simulink model "hmag_ctrl_with_hcomp_2021_09_27"  (R2020a)
settings: Solver=ode23tb  StartTime=0.0  StopTime=simlength  MaxStep=Ts
values from neighbouring files (symbols this model uses):
  Afd = [exp(-Ts*w)*(1+Ts*w) exp(-Ts*w)*Ts; -exp(-Ts*w)*Ts*w^2 exp(-Ts*w)*(1-Ts*w)]    [init_2021_09_27.m]
  Afd_res = [exp(-Ts*wres)*(1+Ts*wres) exp(-Ts*wres)*Ts; -exp(-Ts*wres)*Ts*wres^2 exp(-Ts*wres)*(1-Ts*wres)]    [init_2021_09_27.m]
  Ares = 1    [init_2021_09_27.m]
  Bfd = [(1-exp(-Ts*w)*(1+Ts*w))/w^2 exp(-Ts*w)*Ts]'    [init_2021_09_27.m]
  Bfd_res = [(1-exp(-Ts*wres)*(1+Ts*wres))/wres^2 exp(-Ts*wres)*Ts]'    [init_2021_09_27.m]
  Cf = [2*w^2 0]    [init_2021_09_27.m]
  Cf_res = [2*wres^2 0]    [init_2021_09_27.m]
  ki = 2    [init_2021_09_27.m]
  ki_comp = 2e-1    (= 0.2)    [init_2021_09_27.m]
  kp = 1    [init_2021_09_27.m]
  kp_comp = 1e-1    (= 0.1)    [init_2021_09_27.m]
  pll_i1 = 2*pi/wres    (= 0.00507614213198)    [init_2021_09_27.m]
  pll_p = 2*pi/wres    (= 0.00507614213198)    [init_2021_09_27.m]
  q1kalman = Ts*10    (= 0.0005)    [init_2021_09_27.m]
  q1kalman_res = Ts    (= 5e-05)    [init_2021_09_27.m]
  q2kalman = Ts*10    (= 0.0005)    [init_2021_09_27.m]
  q2kalman_res = Ts    (= 5e-05)    [init_2021_09_27.m]
  Rkalman = 1e-2/q1kalman    (= 20)    [init_2021_09_27.m]
  Rkalman_res = 1/Ts    (= 20000)    [init_2021_09_27.m]
  simlength = 50    [init_2021_09_27.m]
  Tc = 1e-5    (= 1e-05)    [init_2021_09_27.m]
  Ts = 1/20e3    (= 5e-05)    [init_2021_09_27.m]
  w = 2*pi*f    (= 314.159265359)    [init_2021_09_27.m]
  wres = 197*2*pi    (= 1237.78750551)    [init_2021_09_27.m]
undefined symbols (not defined in the file or in its folder): magnitude
libraries: simulink x1, cstblocks x1
settings Model: SimulationMode=accelerator  Creator=dbagn  LastModifiedBy=dabagnara
settings SolverCC: SolverResetMethod=Robust
settings DataIOCC: ReturnWorkspaceOutputs=off

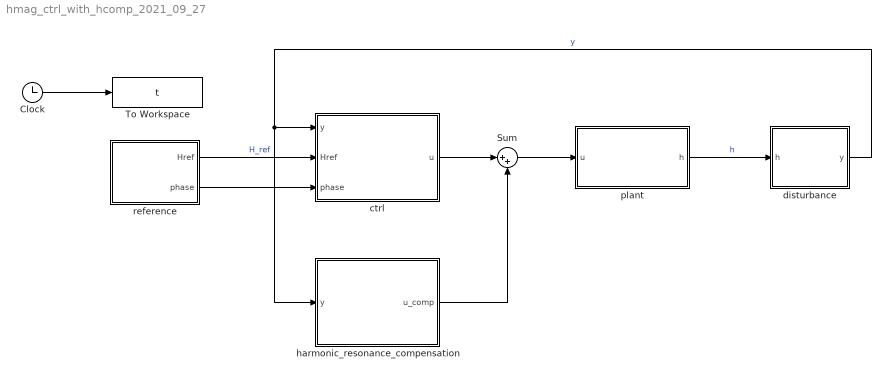
== system hmag_ctrl_with_hcomp_2021_09_27 ==
  Clock : Clock
  Sum : Sum  Inputs=|++
  To Workspace : ToWorkspace  VariableName=t  SampleTime=Tc
      settings: MaxDataPoints=Nc
  ctrl : Subsystem
  disturbance : Subsystem
  harmonic_resonance_compensation : Subsystem
  plant : Subsystem
  reference : Subsystem
  wires:
  reference/1(Href) -> ctrl/2(Href)  "H_ref"
  plant/1(h) -> disturbance/1(h)  "h"
  disturbance/1(y) -> harmonic_resonance_compensation/1(y), ctrl/1(y)  "y"
  reference/2(phase) -> ctrl/3(phase)
  Clock/1 -> To Workspace/1
  ctrl/1(u) -> Sum/1
  Sum/1 -> plant/1(u)
  harmonic_resonance_compensation/1(u_comp) -> Sum/2

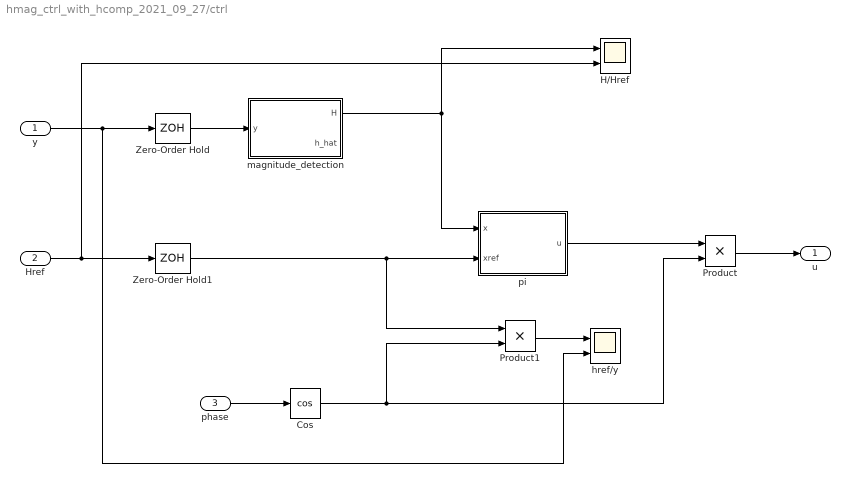
== system hmag_ctrl_with_hcomp_2021_09_27/ctrl ==
  y : Inport
  Href : Inport  Port=2
  phase : Inport  Port=3
  Cos : Trigonometry  Operator=cos
  H/Href : Scope  NumInputPorts=2
  Product : Product
  Product1 : Product
  Zero-Order Hold : ZeroOrderHold  SampleTime=Ts
  Zero-Order Hold1 : ZeroOrderHold  SampleTime=Ts
  href/y : Scope  NumInputPorts=2
  magnitude_detection : Subsystem
  pi : Subsystem  mask{kp=kp, ki=ki, ts=Ts, sat_pos=inf, sat_neg=-inf}
  u : Outport  VectorParamsAs1DForOutWhenUnconnected=off
  wires:
  Href/1 -> H/Href/2, Zero-Order Hold1/1
  y/1 -> href/y/2, Zero-Order Hold/1
  magnitude_detection/1(H) -> H/Href/1, pi/1(x)
  Zero-Order Hold/1 -> magnitude_detection/1(y)
  Zero-Order Hold1/1 -> pi/2(xref), Product1/1
  phase/1 -> Cos/1
  Cos/1 -> Product/2, Product1/2
  Product/1 -> u/1
  Product1/1 -> href/y/1
  pi/1(u) -> Product/1

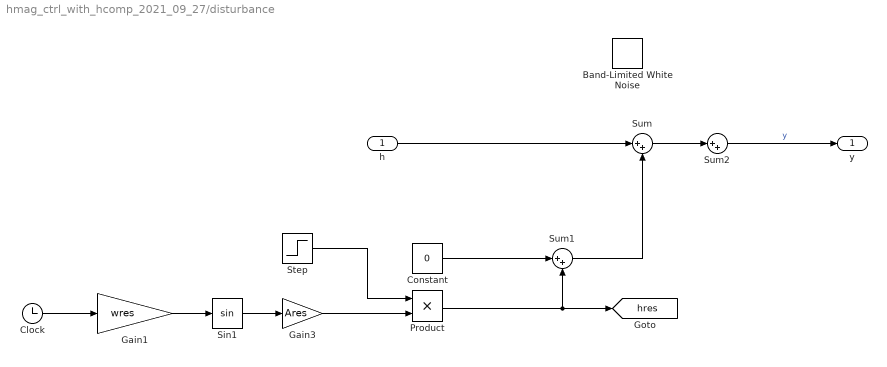
== system hmag_ctrl_with_hcomp_2021_09_27/disturbance ==
  h : Inport
  Band-Limited White Noise : simulink/Sources/Band-Limited White Noise  Cov=Tc  Ts=Tc  seed=[23341]
  Clock : Clock
  Constant : Constant  Value=0
  Gain1 : Gain  Gain=wres
  Gain3 : Gain  Gain=Ares
  Product : Product
  Sin1 : Trigonometry
  Step : Step  Time=simlength/2  Before=1  SampleTime=0
  Sum : Sum  Inputs=|++
  Sum1 : Sum  Inputs=|++
  Sum2 : Sum  Inputs=|++
  y : Outport
  tag scope: hres=global
  wires:
  Sin1/1 -> Gain3/1
  Clock/1 -> Gain1/1
  Sum/1 -> Sum2/1
  Constant/1 -> Sum1/1
  Sum2/1 -> y/1  "y"
  Sum1/1 -> Sum/2
  Gain1/1 -> Sin1/1
  h/1 -> Sum/1
  Gain3/1 -> Product/2
  Step/1 -> Product/1
  Product/1 -> Sum1/2, [hres]

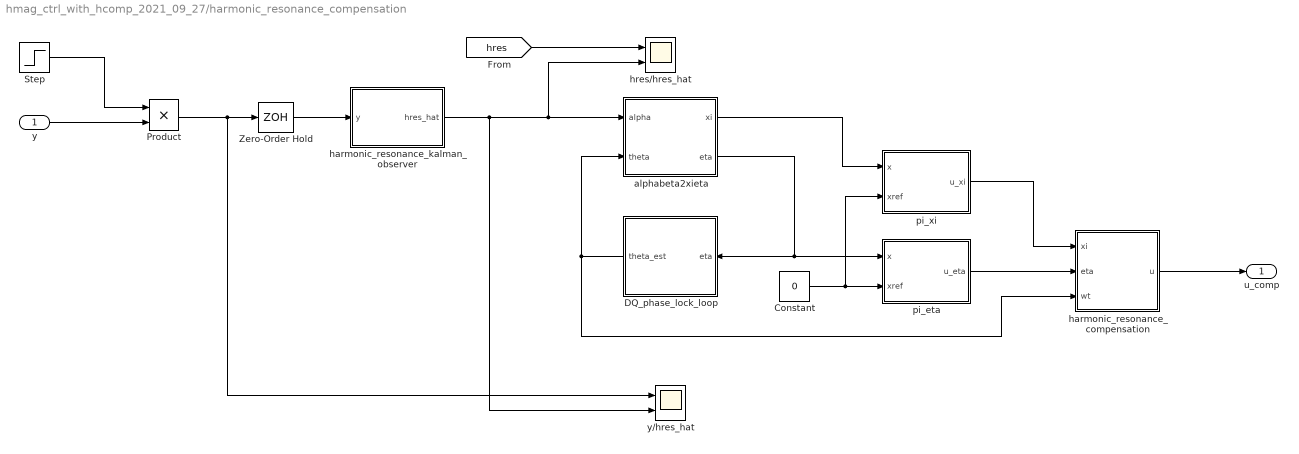
== system hmag_ctrl_with_hcomp_2021_09_27/harmonic_resonance_compensation ==
  y : Inport
  Constant : Constant  Value=0
  DQ_phase_lock_loop : Subsystem
  Product : Product
  Step : Step  Time=simlength/2  SampleTime=0
  Zero-Order Hold : ZeroOrderHold  SampleTime=Ts
  alphabeta2xieta : Subsystem
  harmonic_resonance_compensation : Subsystem
  harmonic_resonance_kalman_observer : Subsystem
  hres/hres_hat : Scope  NumInputPorts=2
  "pi_eta " : Subsystem  mask{kp=kp_comp, ki=ki_comp, ts=Ts, sat_pos=inf, sat_neg=-inf}
  pi_xi : Subsystem  mask{kp=kp_comp, ki=ki_comp, ts=Ts, sat_pos=inf, sat_neg=-inf}
  y/hres_hat : Scope  NumInputPorts=2
  u_comp : Outport  VectorParamsAs1DForOutWhenUnconnected=off
  wires:
  Zero-Order Hold/1 -> harmonic_resonance_kalman_observer/1(y)
  Constant/1 -> pi_xi/2(xref), "pi_eta "/2(xref)
  harmonic_resonance_kalman_observer/1(hres_hat) -> y/hres_hat/2, hres/hres_hat/2, alphabeta2xieta/1(alpha)
  pi_xi/1(u_xi) -> harmonic_resonance_compensation/1(xi)
  "pi_eta "/1(u_eta) -> harmonic_resonance_compensation/2(eta)
  alphabeta2xieta/2(eta) -> "pi_eta "/1(x), DQ_phase_lock_loop/1(eta)
  DQ_phase_lock_loop/1(theta_est) -> harmonic_resonance_compensation/3(wt), alphabeta2xieta/2(theta)
  alphabeta2xieta/1(xi) -> pi_xi/1(x)
  [hres] -> hres/hres_hat/1
  harmonic_resonance_compensation/1(u) -> u_comp/1
  Step/1 -> Product/1
  y/1 -> Product/2
  Product/1 -> y/hres_hat/1, Zero-Order Hold/1

== system hmag_ctrl_with_hcomp_2021_09_27/plant ==
  u : Inport
  LTI System : cstblocks/LTI System  sys=plant  IC=[]
  h : Outport  VectorParamsAs1DForOutWhenUnconnected=off
  wires:
  LTI System/1 -> h/1
  u/1 -> LTI System/1

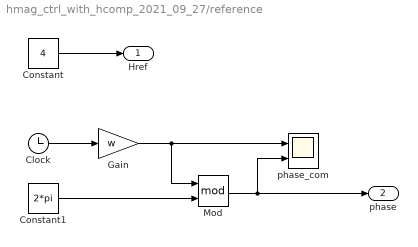
== system hmag_ctrl_with_hcomp_2021_09_27/reference ==
  Clock : Clock
  Constant : Constant  Value=4
  Constant1 : Constant  Value=2*pi
  Gain : Gain  Gain=w
  Mod : Math  Operator=mod  SaturateOnIntegerOverflow=on
  phase_com : Scope  NumInputPorts=2
  Href : Outport
  phase : Outport  Port=2
  wires:
  Clock/1 -> Gain/1
  Constant/1 -> Href/1
  Constant1/1 -> Mod/2
  Gain/1 -> phase_com/1, Mod/1
  Mod/1 -> phase_com/2, phase/1

== system hmag_ctrl_with_hcomp_2021_09_27/ctrl/magnitude_detection ==
  y : Inport
  Manual Switch : ManualSwitch
  kalman observer : Subsystem  Commented=on
  magnitude_calc : Subsystem
  H : Outport
  h_hat : Outport  Port=2
  wires:
  magnitude_calc/1(a) -> H/1
  y/1 -> Manual Switch/1, kalman observer/1(y)
  Manual Switch/1 -> h_hat/1, magnitude_calc/1(alpha)
  kalman observer/1(h_hat) -> Manual Switch/2

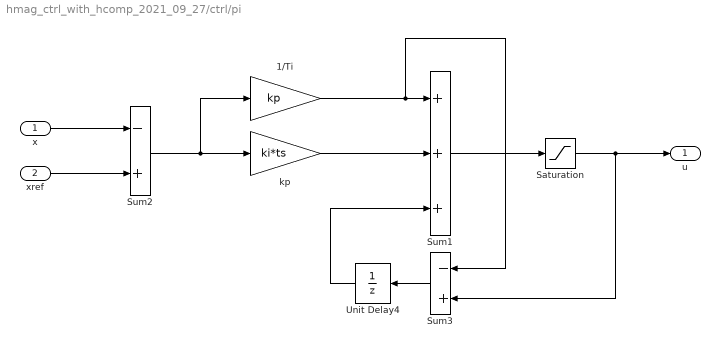
== system hmag_ctrl_with_hcomp_2021_09_27/ctrl/pi ==
  x : Inport
  xref : Inport  Port=2
  1/Ti : Gain  Gain=kp  SaturateOnIntegerOverflow=on  OutDataTypeStr=Inherit: Same as input  ParamDataTypeStr=Inherit: Same as input
  Saturation : Saturate  UpperLimit=sat_pos  LowerLimit=sat_neg
  Sum1 : Sum  Inputs=+++  SaturateOnIntegerOverflow=on
  Sum2 : Sum  Inputs=-+  SaturateOnIntegerOverflow=on
  Sum3 : Sum  Inputs=-+  SaturateOnIntegerOverflow=on
  Unit Delay4 : UnitDelay  SampleTime=ts  HasFrameUpgradeWarning=on
  kp : Gain  Gain=ki*ts  SaturateOnIntegerOverflow=on  OutDataTypeStr=Inherit: Same as input  ParamDataTypeStr=Inherit: Same as input
  u : Outport
  wires:
  xref/1 -> Sum2/2
  kp/1 -> Sum1/2
  Sum2/1 -> kp/1, 1/Ti/1
  1/Ti/1 -> Sum1/1, Sum3/1
  Sum3/1 -> Unit Delay4/1
  x/1 -> Sum2/1
  Sum1/1 -> Saturation/1
  Unit Delay4/1 -> Sum1/3
  Saturation/1 -> u/1, Sum3/2

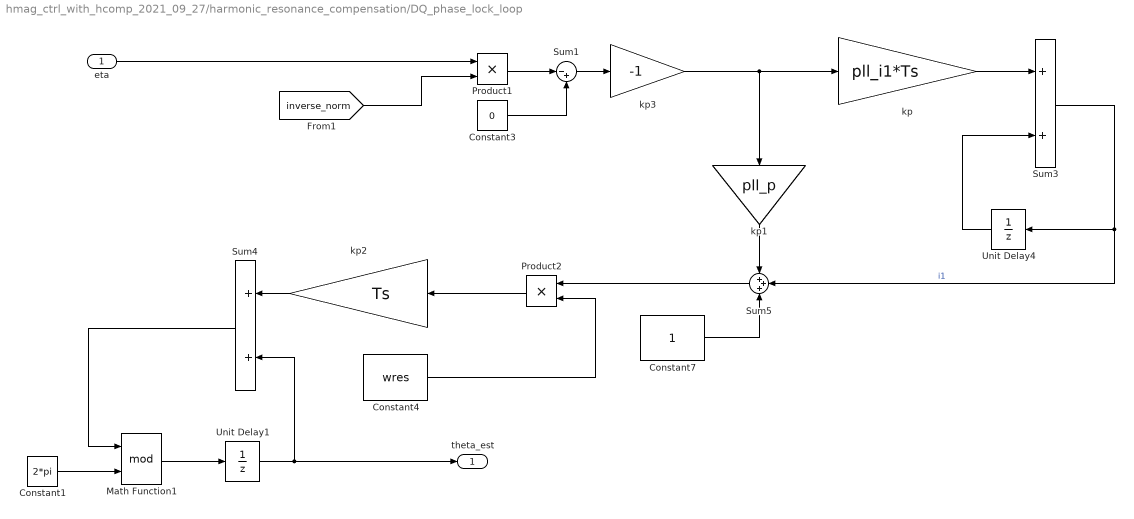
== system hmag_ctrl_with_hcomp_2021_09_27/harmonic_resonance_compensation/DQ_phase_lock_loop ==
  eta : Inport
  Constant1 : Constant  Value=2*pi
  Constant3 : Constant  Value=0
  Constant4 : Constant  Value=wres
  Constant7 : Constant
  Math Function1 : Math  Operator=mod  SignedPower=on  SaturateOnIntegerOverflow=on
  Product1 : Product  RndMeth=Zero
  Product2 : Product  RndMeth=Zero
  Sum1 : Sum  Inputs=|-+
  Sum3 : Sum  SaturateOnIntegerOverflow=on
  Sum4 : Sum  SaturateOnIntegerOverflow=on
  Sum5 : Sum  Inputs=+++
  Unit Delay1 : UnitDelay  SampleTime=Ts  HasFrameUpgradeWarning=on
  Unit Delay4 : UnitDelay  SampleTime=Ts  HasFrameUpgradeWarning=on
  kp : Gain  Gain=pll_i1*Ts  SaturateOnIntegerOverflow=on  OutDataTypeStr=Inherit: Same as input  ParamDataTypeStr=Inherit: Same as input
  kp1 : Gain  Gain=pll_p  SaturateOnIntegerOverflow=on  OutDataTypeStr=Inherit: Same as input  ParamDataTypeStr=Inherit: Same as input
  kp2 : Gain  Gain=Ts  SaturateOnIntegerOverflow=on  OutDataTypeStr=Inherit: Same as input  ParamDataTypeStr=Inherit: Same as input
  kp3 : Gain  Gain=-1  SaturateOnIntegerOverflow=on  OutDataTypeStr=Inherit: Same as input  ParamDataTypeStr=Inherit: Same as input
  theta_est : Outport  VectorParamsAs1DForOutWhenUnconnected=off
  wires:
  Constant7/1 -> Sum5/3
  Constant3/1 -> Sum1/2
  [inverse_norm] -> Product1/2
  Product2/1 -> kp2/1
  kp/1 -> Sum3/1
  Sum4/1 -> Math Function1/1
  kp1/1 -> Sum5/1
  Product1/1 -> Sum1/1
  Sum1/1 -> kp3/1
  Unit Delay1/1 -> theta_est/1, Sum4/2
  Sum3/1 -> Sum5/2, Unit Delay4/1  "i1"
  Unit Delay4/1 -> Sum3/2
  kp2/1 -> Sum4/1
  Sum5/1 -> Product2/1
  Constant4/1 -> Product2/2
  Math Function1/1 -> Unit Delay1/1
  Constant1/1 -> Math Function1/2
  kp3/1 -> kp/1, kp1/1
  eta/1 -> Product1/1

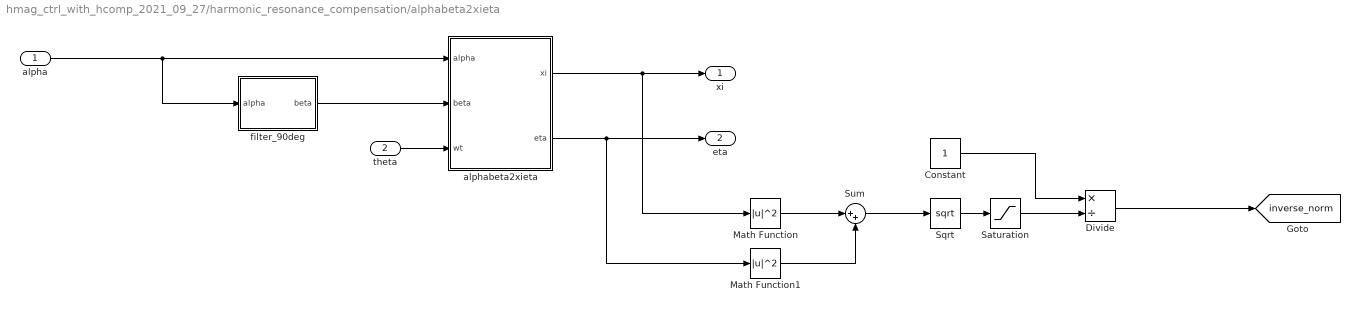
== system hmag_ctrl_with_hcomp_2021_09_27/harmonic_resonance_compensation/alphabeta2xieta ==
  alpha : Inport
  theta : Inport  Port=2
  Constant : Constant
  Divide : Product  Inputs=*/
  Math Function : Math  Operator=magnitude^2  SaturateOnIntegerOverflow=on
  Math Function1 : Math  Operator=magnitude^2  SaturateOnIntegerOverflow=on
  Saturation : Saturate  UpperLimit=inf  LowerLimit=1e-2
  Sqrt : Sqrt  SaturateOnIntegerOverflow=on
  Sum : Sum  Inputs=|++
  alphabeta2xieta : Subsystem
  filter_90deg : Subsystem
  xi : Outport
  eta : Outport  Port=2
  tag scope: inverse_norm=global
  wires:
  alpha/1 -> alphabeta2xieta/1(alpha), filter_90deg/1(alpha)
  filter_90deg/1(beta) -> alphabeta2xieta/2(beta)
  theta/1 -> alphabeta2xieta/3(wt)
  alphabeta2xieta/1(xi) -> xi/1, Math Function/1
  alphabeta2xieta/2(eta) -> Math Function1/1, eta/1
  Math Function/1 -> Sum/1
  Math Function1/1 -> Sum/2
  Sum/1 -> Sqrt/1
  Divide/1 -> [inverse_norm]
  Constant/1 -> Divide/1
  Sqrt/1 -> Saturation/1
  Saturation/1 -> Divide/2

== system hmag_ctrl_with_hcomp_2021_09_27/harmonic_resonance_compensation/harmonic_resonance_compensation ==
  xi : Inport
  eta : Inport  Port=2
  wt : Inport  Port=3
  xieta2alphabeta : Subsystem
  u : Outport  VectorParamsAs1DForOutWhenUnconnected=off
  wires:
  xi/1 -> xieta2alphabeta/1(xi)
  eta/1 -> xieta2alphabeta/2(eta)
  wt/1 -> xieta2alphabeta/3(wt)
  xieta2alphabeta/1(alpha) -> u/1

== system hmag_ctrl_with_hcomp_2021_09_27/harmonic_resonance_compensation/harmonic_resonance_kalman_observer ==
  y : Inport
  Constant2 : Constant  Value=wres
  Constant3 : Constant  Value=q1kalman_res
  Constant4 : Constant  Value=q2kalman_res
  Constant5 : Constant  Value=Rkalman_res
  Constant6 : Constant  Value=Ts
  harmonic_resonance_kalman_observer : MATLAB Function  TreatAsAtomicUnit=on  SystemSampleTime=Ts
  hres_hat : Outport
  wires:
  Constant2/1 -> harmonic_resonance_kalman_observer/2(w)
  y/1 -> harmonic_resonance_kalman_observer/1(y)
  Constant6/1 -> harmonic_resonance_kalman_observer/3(Ts)
  Constant5/1 -> harmonic_resonance_kalman_observer/6(r)
  Constant3/1 -> harmonic_resonance_kalman_observer/4(q1)
  Constant4/1 -> harmonic_resonance_kalman_observer/5(q2)
  harmonic_resonance_kalman_observer/1(h_hat) -> hres_hat/1

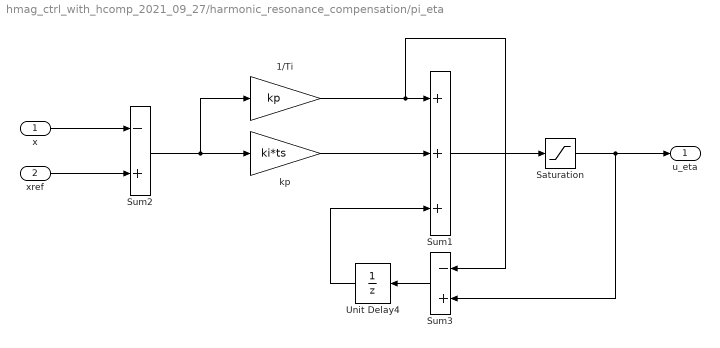
== system hmag_ctrl_with_hcomp_2021_09_27/harmonic_resonance_compensation/pi_eta  ==
  x : Inport
  xref : Inport  Port=2
  1/Ti : Gain  Gain=kp  SaturateOnIntegerOverflow=on  OutDataTypeStr=Inherit: Same as input  ParamDataTypeStr=Inherit: Same as input
  Saturation : Saturate  UpperLimit=sat_pos  LowerLimit=sat_neg
  Sum1 : Sum  Inputs=+++  SaturateOnIntegerOverflow=on
  Sum2 : Sum  Inputs=-+  SaturateOnIntegerOverflow=on
  Sum3 : Sum  Inputs=-+  SaturateOnIntegerOverflow=on
  Unit Delay4 : UnitDelay  SampleTime=ts  HasFrameUpgradeWarning=on
  kp : Gain  Gain=ki*ts  SaturateOnIntegerOverflow=on  OutDataTypeStr=Inherit: Same as input  ParamDataTypeStr=Inherit: Same as input
  u_eta : Outport
  wires:
  Saturation/1 -> Sum3/2, u_eta/1
  Unit Delay4/1 -> Sum1/3
  Sum1/1 -> Saturation/1
  x/1 -> Sum2/1
  Sum3/1 -> Unit Delay4/1
  1/Ti/1 -> Sum3/1, Sum1/1
  Sum2/1 -> 1/Ti/1, kp/1
  kp/1 -> Sum1/2
  xref/1 -> Sum2/2

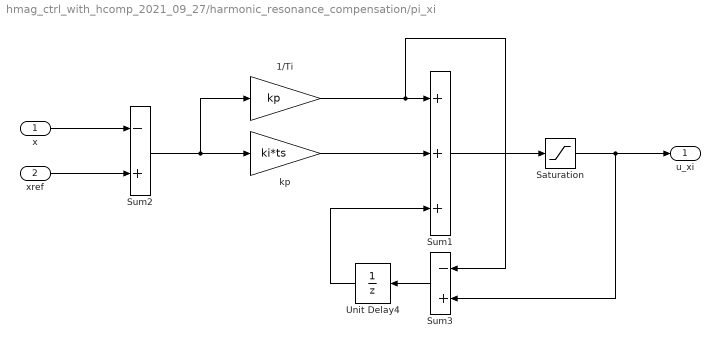
== system hmag_ctrl_with_hcomp_2021_09_27/harmonic_resonance_compensation/pi_xi ==
  x : Inport
  xref : Inport  Port=2
  1/Ti : Gain  Gain=kp  SaturateOnIntegerOverflow=on  OutDataTypeStr=Inherit: Same as input  ParamDataTypeStr=Inherit: Same as input
  Saturation : Saturate  UpperLimit=sat_pos  LowerLimit=sat_neg
  Sum1 : Sum  Inputs=+++  SaturateOnIntegerOverflow=on
  Sum2 : Sum  Inputs=-+  SaturateOnIntegerOverflow=on
  Sum3 : Sum  Inputs=-+  SaturateOnIntegerOverflow=on
  Unit Delay4 : UnitDelay  SampleTime=ts  HasFrameUpgradeWarning=on
  kp : Gain  Gain=ki*ts  SaturateOnIntegerOverflow=on  OutDataTypeStr=Inherit: Same as input  ParamDataTypeStr=Inherit: Same as input
  u_xi : Outport
  wires:
  xref/1 -> Sum2/2
  kp/1 -> Sum1/2
  Sum2/1 -> kp/1, 1/Ti/1
  1/Ti/1 -> Sum1/1, Sum3/1
  Sum3/1 -> Unit Delay4/1
  x/1 -> Sum2/1
  Sum1/1 -> Saturation/1
  Unit Delay4/1 -> Sum1/3
  Saturation/1 -> u_xi/1, Sum3/2

== system hmag_ctrl_with_hcomp_2021_09_27/ctrl/magnitude_detection/kalman observer ==
  y : Inport
  Constant2 : Constant  Value=w
  Constant3 : Constant  Value=q1kalman
  Constant4 : Constant  Value=q2kalman
  Constant5 : Constant  Value=Rkalman
  Constant6 : Constant  Value=Ts
  kalman_observer : MATLAB Function  TreatAsAtomicUnit=on  SystemSampleTime=Ts
  h_hat : Outport
  wires:
  y/1 -> kalman_observer/1(y)
  Constant2/1 -> kalman_observer/2(w)
  kalman_observer/1(h_hat) -> h_hat/1
  Constant6/1 -> kalman_observer/3(Ts)
  Constant5/1 -> kalman_observer/6(r)
  Constant3/1 -> kalman_observer/4(q1)
  Constant4/1 -> kalman_observer/5(q2)

== system hmag_ctrl_with_hcomp_2021_09_27/ctrl/magnitude_detection/magnitude_calc ==
  alpha : Inport
  filter_90deg : Subsystem
  magnitude : Subsystem
  a : Outport
  wires:
  magnitude/1(a) -> a/1
  alpha/1 -> filter_90deg/1(u), magnitude/1(alpha)  "cos"
  filter_90deg/1(y) -> magnitude/2(beta)  "sin"

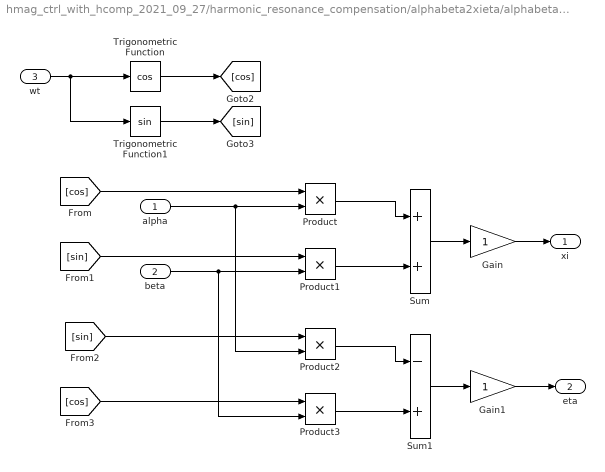
== system hmag_ctrl_with_hcomp_2021_09_27/harmonic_resonance_compensation/alphabeta2xieta/alphabeta2xieta ==
  alpha : Inport
  beta : Inport  Port=2
  wt : Inport  Port=3
  Gain : Gain
  Gain1 : Gain
  Product{,1..3} (4 alike) : Product  RndMeth=Zero
  Sum : Sum
  Sum1 : Sum  Inputs=-+
  Trigonometric Function : Trigonometry  Operator=cos
  Trigonometric Function1 : Trigonometry
  xi : Outport  VectorParamsAs1DForOutWhenUnconnected=off
  eta : Outport  Port=2  VectorParamsAs1DForOutWhenUnconnected=off
  wires:
  wt/1 -> Trigonometric Function1/1, Trigonometric Function/1
  Trigonometric Function/1 -> [cos]
  Trigonometric Function1/1 -> [sin]
  Gain1/1 -> eta/1
  Gain/1 -> xi/1
  Sum1/1 -> Gain1/1
  [cos] -> Product3/1
  Product3/1 -> Sum1/2
  Product2/1 -> Sum1/1
  [sin] -> Product2/1
  Sum/1 -> Gain/1
  beta/1 -> Product1/2, Product3/2
  [sin] -> Product1/1
  Product1/1 -> Sum/2
  Product/1 -> Sum/1
  alpha/1 -> Product2/2, Product/2
  [cos] -> Product/1

== system hmag_ctrl_with_hcomp_2021_09_27/harmonic_resonance_compensation/alphabeta2xieta/filter_90deg ==
  alpha : Inport
  Sum5 : Sum  Inputs=|++
  Unit Delay4 : UnitDelay  SampleTime=Ts  HasFrameUpgradeWarning=on
  kp1 : Gain  Gain=Bfd_res  Multiplication=Matrix(K*u)  SaturateOnIntegerOverflow=on  OutDataTypeStr=Inherit: Same as input  ParamDataTypeStr=Inherit: Same as input
  kp2 : Gain  Gain=Afd_res  Multiplication=Matrix(K*u)  SaturateOnIntegerOverflow=on  OutDataTypeStr=Inherit: Same as input  ParamDataTypeStr=Inherit: Same as input
  kp3 : Gain  Gain=Cf_res  Multiplication=Matrix(K*u)  SaturateOnIntegerOverflow=on  OutDataTypeStr=Inherit: Same as input  ParamDataTypeStr=Inherit: Same as input
  beta : Outport
  wires:
  Unit Delay4/1 -> kp2/1, kp3/1
  Sum5/1 -> Unit Delay4/1
  kp3/1 -> beta/1
  kp2/1 -> Sum5/2
  kp1/1 -> Sum5/1
  alpha/1 -> kp1/1

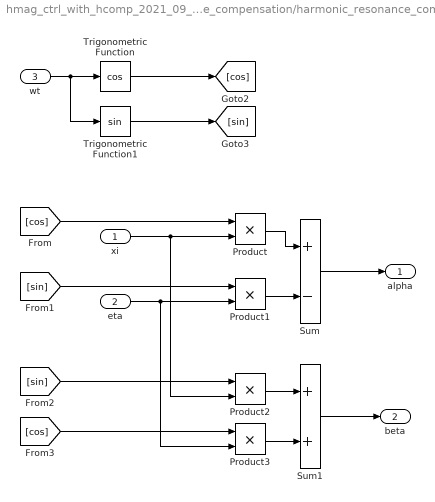
== system hmag_ctrl_with_hcomp_2021_09_27/harmonic_resonance_compensation/harmonic_resonance_compensation/xieta2alphabeta ==
  xi : Inport
  eta : Inport  Port=2
  wt : Inport  Port=3
  Product{,1..3} (4 alike) : Product  RndMeth=Zero
  Sum : Sum  Inputs=+-
  Sum1 : Sum
  Trigonometric Function : Trigonometry  Operator=cos
  Trigonometric Function1 : Trigonometry
  alpha : Outport  VectorParamsAs1DForOutWhenUnconnected=off
  beta : Outport  Port=2  VectorParamsAs1DForOutWhenUnconnected=off
  wires:
  Sum1/1 -> beta/1
  [cos] -> Product3/1
  Product3/1 -> Sum1/2
  Product2/1 -> Sum1/1
  [sin] -> Product2/1
  Sum/1 -> alpha/1
  eta/1 -> Product3/2, Product1/2
  [sin] -> Product1/1
  Product1/1 -> Sum/2
  Product/1 -> Sum/1
  xi/1 -> Product2/2, Product/2
  [cos] -> Product/1
  Trigonometric Function1/1 -> [sin]
  Trigonometric Function/1 -> [cos]
  wt/1 -> Trigonometric Function/1, Trigonometric Function1/1

== system hmag_ctrl_with_hcomp_2021_09_27/ctrl/magnitude_detection/magnitude_calc/filter_90deg ==
  u : Inport
  Sum5 : Sum  Inputs=|++
  Unit Delay4 : UnitDelay  SampleTime=Ts  HasFrameUpgradeWarning=on
  kp1 : Gain  Gain=Bfd  Multiplication=Matrix(K*u)  SaturateOnIntegerOverflow=on  OutDataTypeStr=Inherit: Same as input  ParamDataTypeStr=Inherit: Same as input
  kp2 : Gain  Gain=Afd  Multiplication=Matrix(K*u)  SaturateOnIntegerOverflow=on  OutDataTypeStr=Inherit: Same as input  ParamDataTypeStr=Inherit: Same as input
  kp3 : Gain  Gain=Cf  Multiplication=Matrix(K*u)  SaturateOnIntegerOverflow=on  OutDataTypeStr=Inherit: Same as input  ParamDataTypeStr=Inherit: Same as input
  y : Outport
  wires:
  Unit Delay4/1 -> kp2/1, kp3/1
  Sum5/1 -> Unit Delay4/1
  kp3/1 -> y/1
  kp2/1 -> Sum5/2
  kp1/1 -> Sum5/1
  u/1 -> kp1/1

== system hmag_ctrl_with_hcomp_2021_09_27/ctrl/magnitude_detection/magnitude_calc/magnitude ==
  alpha : Inport
  beta : Inport  Port=2
  Math Function : Math  Operator=magnitude^2  SaturateOnIntegerOverflow=on
  Math Function1 : Math  Operator=magnitude^2  SaturateOnIntegerOverflow=on
  Sqrt : Sqrt  SaturateOnIntegerOverflow=on
  Sum : Sum  Inputs=|++
  a : Outport
  wires:
  alpha/1 -> Math Function/1
  beta/1 -> Math Function1/1
  Math Function/1 -> Sum/1
  Math Function1/1 -> Sum/2
  Sum/1 -> Sqrt/1
  Sqrt/1 -> a/1

== matlab function hmag_ctrl_with_hcomp_2021_09_27/ctrl/magnitude_detection/kalman observer/kalman_observer ==
  data: y input; h_hat output; w input; Ts input; q1 input; q2 input; r input
function h_hat   = KFO(y,w,Ts,q1,q2,r)

    persistent   x1_po x2_po p11_po p12_po p21_po p22_po

    if isempty(x1_po)
        x1_po = 0;
        x2_po = 0;
        p11_po = 0;
        p12_po = 0;
        p21_po = 0;
        p22_po = 0;        
    end
    
    a11 = cos(w*Ts);
    a12 = sin(w*Ts);
    a21 = -sin(w*Ts);
    a22 = cos(w*Ts);
   
    
    
    x1_pr = a11*x1_po + a12*x2_po;
    x2_pr = a21*x1_po + a22*x2_po;
    
    p11_pr = q1 + a11*(a11*p11_po+a12*p21_po) + a12*(a11*p12_po+a12*p22_po);
    p12_pr = a21*(a11*p11_po+a12*p21_po) + a22*(a11*p12_po+a12*p22_po);
    p21_pr = a11*(a21*p11_po+a22*p21_po) + a12*(a21*p12_po+a22*p22_po);
    p22_pr = q2 + a21*(a21*p11_po+a22*p21_po) + a22*(a21*p12_po+a22*p22_po);
    
    l1 = p11_pr/(p11_pr + r);
    l2 = p21_pr/(p11_pr + r);
    
    x1_po = x1_pr + l1*(y-x1_pr);
    x2_po = x2_pr + l2*(y-x1_pr);
    
    p11_po = (1-l1)*p11_pr;
    p12_po = (1-l1)*p12_pr;
    p21_po = p21_pr-l2*p11_pr;
    p22_po = p22_pr-l2*p12_pr;
    
    
    
    h_hat = x1_pr;
end

== matlab function hmag_ctrl_with_hcomp_2021_09_27/harmonic_resonance_compensation/harmonic_resonance_kalman_observer/harmonic_resonance_kalman_observer ==
  data: y input; h_hat output; w input; Ts input; q1 input; q2 input; r input
function h_hat   = KFO(y,w,Ts,q1,q2,r)

    persistent   x1_po x2_po p11_po p12_po p21_po p22_po

    if isempty(x1_po)
        x1_po = 0;
        x2_po = 0;
        p11_po = 0;
        p12_po = 0;
        p21_po = 0;
        p22_po = 0;        
    end
    
    a11 = cos(w*Ts);
    a12 = sin(w*Ts);
    a21 = -sin(w*Ts);
    a22 = cos(w*Ts);
   
    
    
    x1_pr = a11*x1_po + a12*x2_po;
    x2_pr = a21*x1_po + a22*x2_po;
    
    p11_pr = q1 + a11*(a11*p11_po+a12*p21_po) + a12*(a11*p12_po+a12*p22_po);
    p12_pr = a21*(a11*p11_po+a12*p21_po) + a22*(a11*p12_po+a12*p22_po);
    p21_pr = a11*(a21*p11_po+a22*p21_po) + a12*(a21*p12_po+a22*p22_po);
    p22_pr = q2 + a21*(a21*p11_po+a22*p21_po) + a22*(a21*p12_po+a22*p22_po);
    
    l1 = p11_pr/(p11_pr + r);
    l2 = p21_pr/(p11_pr + r);
    
    x1_po = x1_pr + l1*(y-x1_pr);
    x2_po = x2_pr + l2*(y-x1_pr);
    
    p11_po = (1-l1)*p11_pr;
    p12_po = (1-l1)*p12_pr;
    p21_po = p21_pr-l2*p11_pr;
    p22_po = p22_pr-l2*p12_pr;
    
    
    
    h_hat = x1_pr;
end
